simulink library "VIS_LIB"  (Simulink 8.6)
settings: Solver=ode45  StartTime=0.0  StopTime=10.0  RelTol=1e-3
undefined symbols (not defined in the file): AC, SIXOSEM_F_WD_AC_MASTER
libraries: cdsFilt x376, cdsEpicsOut x253, cdsEpicsIn x179, cdsTP x123, VIS_LIB x95, cdsMuxMatrix x91, cdsEpicsStringIn x75, cdsFiltCtrl x72, cdsFunctionCall x70, cdsRms x59, KAGRA_UTIL x25, STATE_BIO_MASTER x5
(part 26 of 38)

== system VIS_LIB/UTILs/OL ==
  note: #DAQ Channels
      |
      | VER_OUT 256
      | HOR_OUT 256
      | SUM_OUT 256
      | CROSS_OUT 256
  SEG1_in : Inport
  SEG2_in : Inport  Port=2
  SEG3_in : Inport  Port=3
  SEG4_in : Inport  Port=4
  CROSS : cdsFilt/Subsystem  Tag=cdsFilt  Description=|
      | Purpose:                                                                                                                                                                                                                                  
      | Standard CDS IIR filter module.                                                                                                                                                                                                           
      |                                                                                                                                                                                                                                           
      | Operation:                                                                                                                                                                                                                                
      | Consists of 10 second order section IIR filters, plus a ramped gain stage. In FE code, also provides pre-defined test points and excitation channel inputs. The filter coefficients are defined in the LIGO system using the 'foton' tool.
      |                                                                                                                                                                                                                                           
      | Usage:                                                                                                                                                                                                                                    
      | Name the part with the desired filter module name.
      settings: AttributesFormatString=%<Tag>
  Demux : Demux
  HOR : cdsFilt/Subsystem  Tag=cdsFilt  Description=|
      | Purpose:                                                                                                                                                                                                                                  
      | Standard CDS IIR filter module.                                                                                                                                                                                                           
      |                                                                                                                                                                                                                                           
      | Operation:                                                                                                                                                                                                                                
      | Consists of 10 second order section IIR filters, plus a ramped gain stage. In FE code, also provides pre-defined test points and excitation channel inputs. The filter coefficients are defined in the LIGO system using the 'foton' tool.
      |                                                                                                                                                                                                                                           
      | Usage:                                                                                                                                                                                                                                    
      | Name the part with the desired filter module name.
      settings: AttributesFormatString=%<Tag>
  MTRX : cdsMuxMatrix/Subsystem  Tag=cdsMuxMatrix  Description=Any size matrix. Inputs and outputs must be connected using Mux and Demux parts.
      settings: AttributesFormatString=%<Tag>
  MTRX_HOR_OUTMON : cdsEpicsOut/Subsystem  Tag=cdsEpicsOutput  Description=|
      | Purpose:                                          
      | Output a FE signal to an EPICS channel.           
      |                                                   
      | Operation:                                        
      | Takes input value and passes it to EPICS record.  
      |                                                   
      | Usage:                                            
      | Name the part with the desired EPICS rrecord name.
      settings: AttributesFormatString=%<Tag>
  MTRX_VER_OUTMON : cdsEpicsOut/Subsystem  Tag=cdsEpicsOutput  Description=|
      | Purpose:                                          
      | Output a FE signal to an EPICS channel.           
      |                                                   
      | Operation:                                        
      | Takes input value and passes it to EPICS record.  
      |                                                   
      | Usage:                                            
      | Name the part with the desired EPICS rrecord name.
      settings: AttributesFormatString=%<Tag>
  Mux : Mux
  PIT_NORM : Product  Inputs=*/
  SEG1 : cdsFilt/Subsystem  Tag=cdsFilt  Description=|
      | Purpose:                                                                                                                                                                                                                                  
      | Standard CDS IIR filter module.                                                                                                                                                                                                           
      |                                                                                                                                                                                                                                           
      | Operation:                                                                                                                                                                                                                                
      | Consists of 10 second order section IIR filters, plus a ramped gain stage. In FE code, also provides pre-defined test points and excitation channel inputs. The filter coefficients are defined in the LIGO system using the 'foton' tool.
      |                                                                                                                                                                                                                                           
      | Usage:                                                                                                                                                                                                                                    
      | Name the part with the desired filter module name.
      settings: AttributesFormatString=%<Tag>
  SEG2 : cdsFilt/Subsystem  Tag=cdsFilt  Description=|
      | Purpose:                                                                                                                                                                                                                                  
      | Standard CDS IIR filter module.                                                                                                                                                                                                           
      |                                                                                                                                                                                                                                           
      | Operation:                                                                                                                                                                                                                                
      | Consists of 10 second order section IIR filters, plus a ramped gain stage. In FE code, also provides pre-defined test points and excitation channel inputs. The filter coefficients are defined in the LIGO system using the 'foton' tool.
      |                                                                                                                                                                                                                                           
      | Usage:                                                                                                                                                                                                                                    
      | Name the part with the desired filter module name.
      settings: AttributesFormatString=%<Tag>
  SEG3 : cdsFilt/Subsystem  Tag=cdsFilt  Description=|
      | Purpose:                                                                                                                                                                                                                                  
      | Standard CDS IIR filter module.                                                                                                                                                                                                           
      |                                                                                                                                                                                                                                           
      | Operation:                                                                                                                                                                                                                                
      | Consists of 10 second order section IIR filters, plus a ramped gain stage. In FE code, also provides pre-defined test points and excitation channel inputs. The filter coefficients are defined in the LIGO system using the 'foton' tool.
      |                                                                                                                                                                                                                                           
      | Usage:                                                                                                                                                                                                                                    
      | Name the part with the desired filter module name.
      settings: AttributesFormatString=%<Tag>
  SEG4 : cdsFilt/Subsystem  Tag=cdsFilt  Description=|
      | Purpose:                                                                                                                                                                                                                                  
      | Standard CDS IIR filter module.                                                                                                                                                                                                           
      |                                                                                                                                                                                                                                           
      | Operation:                                                                                                                                                                                                                                
      | Consists of 10 second order section IIR filters, plus a ramped gain stage. In FE code, also provides pre-defined test points and excitation channel inputs. The filter coefficients are defined in the LIGO system using the 'foton' tool.
      |                                                                                                                                                                                                                                           
      | Usage:                                                                                                                                                                                                                                    
      | Name the part with the desired filter module name.
      settings: AttributesFormatString=%<Tag>
  SUM : cdsFilt/Subsystem  Tag=cdsFilt  Description=|
      | Purpose:                                                                                                                                                                                                                                  
      | Standard CDS IIR filter module.                                                                                                                                                                                                           
      |                                                                                                                                                                                                                                           
      | Operation:                                                                                                                                                                                                                                
      | Consists of 10 second order section IIR filters, plus a ramped gain stage. In FE code, also provides pre-defined test points and excitation channel inputs. The filter coefficients are defined in the LIGO system using the 'foton' tool.
      |                                                                                                                                                                                                                                           
      | Usage:                                                                                                                                                                                                                                    
      | Name the part with the desired filter module name.
      settings: AttributesFormatString=%<Tag>
  Saturation : Saturate  UpperLimit=1e12  LowerLimit=1
  Terminator5 : Terminator
  VER : cdsFilt/Subsystem  Tag=cdsFilt  Description=|
      | Purpose:                                                                                                                                                                                                                                  
      | Standard CDS IIR filter module.                                                                                                                                                                                                           
      |                                                                                                                                                                                                                                           
      | Operation:                                                                                                                                                                                                                                
      | Consists of 10 second order section IIR filters, plus a ramped gain stage. In FE code, also provides pre-defined test points and excitation channel inputs. The filter coefficients are defined in the LIGO system using the 'foton' tool.
      |                                                                                                                                                                                                                                           
      | Usage:                                                                                                                                                                                                                                    
      | Name the part with the desired filter module name.
      settings: AttributesFormatString=%<Tag>
  YAW_NORM : Product  Inputs=*/
  V : Outport
  H : Outport  Port=2
  wires:
  SEG4_in/1 -> SEG4/1
  SEG3_in/1 -> SEG3/1
  SEG1_in/1 -> SEG1/1
  SEG2_in/1 -> SEG2/1
  Mux/1 -> MTRX/1
  MTRX/1 -> Demux/1
  SEG1/1 -> Mux/1
  SEG2/1 -> Mux/2
  SEG3/1 -> Mux/3
  SEG4/1 -> Mux/4
  VER/1 -> V/1
  HOR/1 -> H/1
  SUM/1 -> Saturation/1
  PIT_NORM/1 -> VER/1
  YAW_NORM/1 -> HOR/1
  Demux/1 -> MTRX_VER_OUTMON/1
  Demux/3 -> SUM/1
  Demux/2 -> MTRX_HOR_OUTMON/1
  Saturation/1 -> PIT_NORM/2, YAW_NORM/2
  MTRX_VER_OUTMON/1 -> PIT_NORM/1
  MTRX_HOR_OUTMON/1 -> YAW_NORM/1
  Demux/4 -> CROSS/1
  CROSS/1 -> Terminator5/1

== system VIS_LIB/UTILs/PAY_6DoF ==
  MNL : Inport
  MNT : Inport  Port=2
  MNV : Inport  Port=3
  MNR : Inport  Port=4
  MNP : Inport  Port=5
  MNY : Inport  Port=6
  IML : Inport  Port=7
  IMT : Inport  Port=8
  IMV : Inport  Port=9
  IMR : Inport  Port=10
  IMP : Inport  Port=11
  IMY : Inport  Port=12
  TML : Inport  Port=13
  TMT : Inport  Port=14
  TMV : Inport  Port=15
  TMR : Inport  Port=16
  TMP : Inport  Port=17
  TMY : Inport  Port=18
  IM : VIS_LIB/UTILs/FBs_6DOF
  MN : VIS_LIB/UTILs/FBs_6DOF
  TM : VIS_LIB/UTILs/FBs_6DOF
  MNLo : Outport
  MNTo : Outport  Port=2
  MNVo : Outport  Port=3
  MNRo : Outport  Port=4
  MNPo : Outport  Port=5
  MNYo : Outport  Port=6
  IMLo : Outport  Port=7
  IMTo : Outport  Port=8
  IMVo : Outport  Port=9
  IMRo : Outport  Port=10
  IMPo : Outport  Port=11
  IMYo : Outport  Port=12
  TMLo : Outport  Port=13
  TMTo : Outport  Port=14
  TMVo : Outport  Port=15
  TMRo : Outport  Port=16
  TMPo : Outport  Port=17
  TMYo : Outport  Port=18
  wires:
  TMR/1 -> TM/4
  TMV/1 -> TM/3
  TMT/1 -> TM/2
  TMP/1 -> TM/5
  IMV/1 -> IM/3
  IMP/1 -> IM/5
  IML/1 -> IM/1
  TMY/1 -> TM/6
  IMT/1 -> IM/2
  TML/1 -> TM/1
  MNY/1 -> MN/6
  MNR/1 -> MN/4
  MNP/1 -> MN/5
  MNT/1 -> MN/2
  MNL/1 -> MN/1
  MNV/1 -> MN/3
  IMY/1 -> IM/6
  IMR/1 -> IM/4
  MN/1 -> MNLo/1
  MN/2 -> MNTo/1
  MN/3 -> MNVo/1
  MN/4 -> MNRo/1
  MN/5 -> MNPo/1
  MN/6 -> MNYo/1
  IM/1 -> IMLo/1
  IM/2 -> IMTo/1
  IM/3 -> IMVo/1
  IM/4 -> IMRo/1
  IM/5 -> IMPo/1
  IM/6 -> IMYo/1
  TM/1 -> TMLo/1
  TM/2 -> TMTo/1
  TM/3 -> TMVo/1
  TM/4 -> TMRo/1
  TM/5 -> TMPo/1
  TM/6 -> TMYo/1

== system VIS_LIB/UTILs/PAY_6DoF_DQ ==
  MNL : Inport
  MNT : Inport  Port=2
  MNV : Inport  Port=3
  MNR : Inport  Port=4
  MNP : Inport  Port=5
  MNY : Inport  Port=6
  IML : Inport  Port=7
  IMT : Inport  Port=8
  IMV : Inport  Port=9
  IMR : Inport  Port=10
  IMP : Inport  Port=11
  IMY : Inport  Port=12
  TML : Inport  Port=13
  TMT : Inport  Port=14
  TMV : Inport  Port=15
  TMR : Inport  Port=16
  TMP : Inport  Port=17
  TMY : Inport  Port=18
  IM : VIS_LIB/UTILs/FBs_6DOF_DQ
  MN : VIS_LIB/UTILs/FBs_6DOF_DQ
  TM : VIS_LIB/UTILs/FBs_6DOF_DQ
  MNLo : Outport
  MNTo : Outport  Port=2
  MNVo : Outport  Port=3
  MNRo : Outport  Port=4
  MNPo : Outport  Port=5
  MNYo : Outport  Port=6
  IMLo : Outport  Port=7
  IMTo : Outport  Port=8
  IMVo : Outport  Port=9
  IMRo : Outport  Port=10
  IMPo : Outport  Port=11
  IMYo : Outport  Port=12
  TMLo : Outport  Port=13
  TMTo : Outport  Port=14
  TMVo : Outport  Port=15
  TMRo : Outport  Port=16
  TMPo : Outport  Port=17
  TMYo : Outport  Port=18
  wires:
  TMR/1 -> TM/4
  TMV/1 -> TM/3
  TMT/1 -> TM/2
  TMP/1 -> TM/5
  IMV/1 -> IM/3
  IMP/1 -> IM/5
  IML/1 -> IM/1
  TMY/1 -> TM/6
  IMT/1 -> IM/2
  TML/1 -> TM/1
  MNY/1 -> MN/6
  MNR/1 -> MN/4
  MNP/1 -> MN/5
  MNT/1 -> MN/2
  MNL/1 -> MN/1
  MNV/1 -> MN/3
  IMY/1 -> IM/6
  IMR/1 -> IM/4
  MN/1 -> MNLo/1
  MN/2 -> MNTo/1
  MN/3 -> MNVo/1
  MN/4 -> MNRo/1
  MN/5 -> MNPo/1
  MN/6 -> MNYo/1
  IM/1 -> IMLo/1
  IM/2 -> IMTo/1
  IM/3 -> IMVo/1
  IM/4 -> IMRo/1
  IM/5 -> IMPo/1
  IM/6 -> IMYo/1
  TM/1 -> TMLo/1
  TM/2 -> TMTo/1
  TM/3 -> TMVo/1
  TM/4 -> TMRo/1
  TM/5 -> TMPo/1
  TM/6 -> TMYo/1

== system VIS_LIB/UTILs/PAY_COILs_DQ ==
  MNV1i : Inport
  MNV2i : Inport  Port=2
  MNV3i : Inport  Port=3
  MNH1i : Inport  Port=4
  MNH2i : Inport  Port=5
  MNH3i : Inport  Port=6
  IMV1i : Inport  Port=7
  IMV2i : Inport  Port=8
  IMV3i : Inport  Port=9
  IMH1i : Inport  Port=10
  IMH2i : Inport  Port=11
  IMH3i : Inport  Port=12
  TMH1i : Inport  Port=13
  TMH2i : Inport  Port=14
  TMH3i : Inport  Port=15
  TMH4i : Inport  Port=16
  IM : VIS_LIB/UTILs/6COILs_DQ
  MN : VIS_LIB/UTILs/6COILs_DQ
  TM : VIS_LIB/UTILs/4COILs_DQ
  MNV1 : Outport
  MNV2 : Outport  Port=2
  MNV3 : Outport  Port=3
  MNH1 : Outport  Port=4
  MNH2 : Outport  Port=5
  MNH3 : Outport  Port=6
  IMV1 : Outport  Port=7
  IMV2 : Outport  Port=8
  IMV3 : Outport  Port=9
  IMH1 : Outport  Port=10
  IMH2 : Outport  Port=11
  IMH3 : Outport  Port=12
  TMH1 : Outport  Port=13
  TMH2 : Outport  Port=14
  TMH3 : Outport  Port=15
  TMH4 : Outport  Port=16
  wires:
  TMH2i/1 -> TM/2
  TMH1i/1 -> TM/1
  TMH4i/1 -> TM/4
  MNV1i/1 -> MN/1
  MNV3i/1 -> MN/3
  MNV2i/1 -> MN/2
  IMH3i/1 -> IM/6
  IMH2i/1 -> IM/5
  MNH2i/1 -> MN/5
  TMH3i/1 -> TM/3
  MNH3i/1 -> MN/6
  IMV1i/1 -> IM/1
  MNH1i/1 -> MN/4
  IMV3i/1 -> IM/3
  IMV2i/1 -> IM/2
  IMH1i/1 -> IM/4
  MN/1 -> MNV1/1
  MN/2 -> MNV2/1
  MN/3 -> MNV3/1
  MN/4 -> MNH1/1
  MN/5 -> MNH2/1
  MN/6 -> MNH3/1
  IM/1 -> IMV1/1
  IM/2 -> IMV2/1
  IM/3 -> IMV3/1
  IM/4 -> IMH1/1
  IM/5 -> IMH2/1
  IM/6 -> IMH3/1
  TM/1 -> TMH1/1
  TM/2 -> TMH2/1
  TM/3 -> TMH3/1
  TM/4 -> TMH4/1

== system VIS_LIB/WD2/AC ==
  F0_In : Inport
  SF_In : Inport  Port=2
  BF_In : Inport  Port=3
  BANDLIM : Subsystem
  BFRMS : cdsRms/Subsystem  Tag=cdsRms  Description=|
      | Purpose:
      | Calculate an RMS based on the input signal.
      settings: AttributesFormatString=%<Tag>
  BF_RMS : cdsTP/Subsystem  Tag=Test Point
      settings: AttributesFormatString=%<Tag>
  BF_RMSMON : cdsEpicsOut/Subsystem  Tag=cdsEpicsOutput  Description=|
      | Purpose:                                          
      | Output a FE signal to an EPICS channel.           
      |                                                   
      | Operation:                                        
      | Takes input value and passes it to EPICS record.  
      |                                                   
      | Usage:                                            
      | Name the part with the desired EPICS rrecord name.
      settings: AttributesFormatString=%<Tag>
  F0RMS : cdsRms/Subsystem  Tag=cdsRms  Description=|
      | Purpose:
      | Calculate an RMS based on the input signal.
      settings: AttributesFormatString=%<Tag>
  F0_RMS : cdsTP/Subsystem  Tag=Test Point
      settings: AttributesFormatString=%<Tag>
  F0_RMSMON : cdsEpicsOut/Subsystem  Tag=cdsEpicsOutput  Description=|
      | Purpose:                                          
      | Output a FE signal to an EPICS channel.           
      |                                                   
      | Operation:                                        
      | Takes input value and passes it to EPICS record.  
      |                                                   
      | Usage:                                            
      | Name the part with the desired EPICS rrecord name.
      settings: AttributesFormatString=%<Tag>
  Operator1 : RelationalOperator  Operator=>  OutDataTypeStr=boolean
  Operator2 : RelationalOperator  Operator=>  OutDataTypeStr=boolean
  Operator3 : RelationalOperator  Operator=>  OutDataTypeStr=boolean
  RMS_MAX : cdsEpicsIn/Subsystem  Tag=cdsEpicsIn  Description=|
      | Purpose:                                                                              
      | Create an EPICS input channel connection to the FE realtime controls.                 
      |                                                                                       
      | Operation:                                                                            
      | Outputs value from an EPICS ai record. Value is floating point with a precision of 3..
      |                                                                                       
      | Usage:                                                                                
      | Name the part with the desired EPICS channel name.
      settings: AttributesFormatString=%<Tag>
  SFRMS : cdsRms/Subsystem  Tag=cdsRms  Description=|
      | Purpose:
      | Calculate an RMS based on the input signal.
      settings: AttributesFormatString=%<Tag>
  SF_RMS : cdsTP/Subsystem  Tag=Test Point
      settings: AttributesFormatString=%<Tag>
  SF_RMSMON : cdsEpicsOut/Subsystem  Tag=cdsEpicsOutput  Description=|
      | Purpose:                                          
      | Output a FE signal to an EPICS channel.           
      |                                                   
      | Operation:                                        
      | Takes input value and passes it to EPICS record.  
      |                                                   
      | Usage:                                            
      | Name the part with the desired EPICS rrecord name.
      settings: AttributesFormatString=%<Tag>
  Sum1 : Sum  Inputs=+++
  FLAG : Outport
  wires:
  BANDLIM/3(BF_Out) -> BFRMS/1
  BF_In/1 -> BANDLIM/3(BF_In)
  F0RMS/1 -> F0_RMS/1, F0_RMSMON/1
  F0_RMSMON/1 -> Operator1/1
  SF_In/1 -> BANDLIM/2(SF_In)
  F0_In/1 -> BANDLIM/1(F0_In)
  SFRMS/1 -> SF_RMS/1, SF_RMSMON/1
  SF_RMSMON/1 -> Operator2/1
  BFRMS/1 -> BF_RMS/1, BF_RMSMON/1
  BF_RMSMON/1 -> Operator3/1
  BANDLIM/2(SF_Out) -> SFRMS/1
  BANDLIM/1(F0_Out) -> F0RMS/1
  RMS_MAX/1 -> Operator3/2, Operator2/2, Operator1/2
  Operator3/1 -> Sum1/3
  Operator2/1 -> Sum1/2
  Operator1/1 -> Sum1/1
  Sum1/1 -> FLAG/1

== system VIS_LIB/WD3/OSEMAC ==
  V1_In : Inport
  V2_In : Inport  Port=2
  V3_In : Inport  Port=3
  H1_In : Inport  Port=4
  H2_In1 : Inport  Port=5
  H3_In1 : Inport  Port=6
  BANDLIM : Subsystem
  H1RMS : cdsRms/Subsystem  Tag=cdsRms  Description=|
      | Purpose:
      | Calculate an RMS based on the input signal.
      settings: AttributesFormatString=%<Tag>
  H1_RMS : cdsTP/Subsystem  Tag=Test Point
      settings: AttributesFormatString=%<Tag>
  H1_RMSMON : cdsEpicsOut/Subsystem  Tag=cdsEpicsOutput  Description=|
      | Purpose:                                          
      | Output a FE signal to an EPICS channel.           
      |                                                   
      | Operation:                                        
      | Takes input value and passes it to EPICS record.  
      |                                                   
      | Usage:                                            
      | Name the part with the desired EPICS rrecord name.
      settings: AttributesFormatString=%<Tag>
  H2RMS : cdsRms/Subsystem  Tag=cdsRms  Description=|
      | Purpose:
      | Calculate an RMS based on the input signal.
      settings: AttributesFormatString=%<Tag>
  H2_RMS : cdsTP/Subsystem  Tag=Test Point
      settings: AttributesFormatString=%<Tag>
  H2_RMSMON : cdsEpicsOut/Subsystem  Tag=cdsEpicsOutput  Description=|
      | Purpose:                                          
      | Output a FE signal to an EPICS channel.           
      |                                                   
      | Operation:                                        
      | Takes input value and passes it to EPICS record.  
      |                                                   
      | Usage:                                            
      | Name the part with the desired EPICS rrecord name.
      settings: AttributesFormatString=%<Tag>
  H3RMS : cdsRms/Subsystem  Tag=cdsRms  Description=|
      | Purpose:
      | Calculate an RMS based on the input signal.
      settings: AttributesFormatString=%<Tag>
  H3_RMS : cdsTP/Subsystem  Tag=Test Point
      settings: AttributesFormatString=%<Tag>
  H3_RMSMON : cdsEpicsOut/Subsystem  Tag=cdsEpicsOutput  Description=|
      | Purpose:                                          
      | Output a FE signal to an EPICS channel.           
      |                                                   
      | Operation:                                        
      | Takes input value and passes it to EPICS record.  
      |                                                   
      | Usage:                                            
      | Name the part with the desired EPICS rrecord name.
      settings: AttributesFormatString=%<Tag>
  Operator{1,3..6} (5 alike) : RelationalOperator  Operator=>  OutDataTypeStr=boolean
  Operator2 : RelationalOperator  Operator=>  OutDataTypeStr=boolean  ZeroCross=off
  RMS_MAX : cdsEpicsIn/Subsystem  Tag=cdsEpicsIn  Description=|
      | Purpose:                                                                              
      | Create an EPICS input channel connection to the FE realtime controls.                 
      |                                                                                       
      | Operation:                                                                            
      | Outputs value from an EPICS ai record. Value is floating point with a precision of 3..
      |                                                                                       
      | Usage:                                                                                
      | Name the part with the desired EPICS channel name.
      settings: AttributesFormatString=%<Tag>
  Sum1 : Sum  Inputs=++++++
  V1RMS : cdsRms/Subsystem  Tag=cdsRms  Description=|
      | Purpose:
      | Calculate an RMS based on the input signal.
      settings: AttributesFormatString=%<Tag>
  V1_RMS : cdsTP/Subsystem  Tag=Test Point
      settings: AttributesFormatString=%<Tag>
  V1_RMSMON : cdsEpicsOut/Subsystem  Tag=cdsEpicsOutput  Description=|
      | Purpose:                                          
      | Output a FE signal to an EPICS channel.           
      |                                                   
      | Operation:                                        
      | Takes input value and passes it to EPICS record.  
      |                                                   
      | Usage:                                            
      | Name the part with the desired EPICS rrecord name.
      settings: AttributesFormatString=%<Tag>
  V2RMS : cdsRms/Subsystem  Tag=cdsRms  Description=|
      | Purpose:
      | Calculate an RMS based on the input signal.
      settings: AttributesFormatString=%<Tag>
  V2_RMS : cdsTP/Subsystem  Tag=Test Point
      settings: AttributesFormatString=%<Tag>
  V2_RMSMON : cdsEpicsOut/Subsystem  Tag=cdsEpicsOutput  Description=|
      | Purpose:                                          
      | Output a FE signal to an EPICS channel.           
      |                                                   
      | Operation:                                        
      | Takes input value and passes it to EPICS record.  
      |                                                   
      | Usage:                                            
      | Name the part with the desired EPICS rrecord name.
      settings: AttributesFormatString=%<Tag>
  V3RMS : cdsRms/Subsystem  Tag=cdsRms  Description=|
      | Purpose:
      | Calculate an RMS based on the input signal.
      settings: AttributesFormatString=%<Tag>
  V3_RMS : cdsTP/Subsystem  Tag=Test Point
      settings: AttributesFormatString=%<Tag>
  V3_RMSMON : cdsEpicsOut/Subsystem  Tag=cdsEpicsOutput  Description=|
      | Purpose:                                          
      | Output a FE signal to an EPICS channel.           
      |                                                   
      | Operation:                                        
      | Takes input value and passes it to EPICS record.  
      |                                                   
      | Usage:                                            
      | Name the part with the desired EPICS rrecord name.
      settings: AttributesFormatString=%<Tag>
  FLAG : Outport
  wires:
  BANDLIM/6(H3_Out) -> H3RMS/1
  BANDLIM/5(H2_Out) -> H2RMS/1
  BANDLIM/4(H1_Out) -> H1RMS/1
  BANDLIM/3(V3_Out) -> V3RMS/1
  BANDLIM/2(V2_Out) -> V2RMS/1
  BANDLIM/1(V1_Out) -> V1RMS/1
  H3_In1/1 -> BANDLIM/6(H3_In)
  H2_In1/1 -> BANDLIM/5(H2_In)
  H1_In/1 -> BANDLIM/4(H1_In)
  V3_In/1 -> BANDLIM/3(V3_In)
  V2_In/1 -> BANDLIM/2(V2_In)
  V1_In/1 -> BANDLIM/1(V1_In)
  Operator1/1 -> Sum1/1
  Operator2/1 -> Sum1/2
  Operator3/1 -> Sum1/3
  Operator4/1 -> Sum1/4
  RMS_MAX/1 -> Operator1/2, Operator2/2, Operator3/2, Operator4/2, Operator5/2, Operator6/2
  V2RMS/1 -> V2_RMS/1, V2_RMSMON/1
  V1RMS/1 -> V1_RMS/1, V1_RMSMON/1
  V3RMS/1 -> V3_RMS/1, V3_RMSMON/1
  H1RMS/1 -> H1_RMS/1, H1_RMSMON/1
  Sum1/1 -> FLAG/1
  H2RMS/1 -> H2_RMS/1, H2_RMSMON/1
  H3RMS/1 -> H3_RMS/1, H3_RMSMON/1
  V1_RMSMON/1 -> Operator1/1
  V2_RMSMON/1 -> Operator2/1
  V3_RMSMON/1 -> Operator3/1
  H1_RMSMON/1 -> Operator4/1
  H2_RMSMON/1 -> Operator5/1
  H3_RMSMON/1 -> Operator6/1
  Operator5/1 -> Sum1/5
  Operator6/1 -> Sum1/6

== system VIS_LIB/WD4/AC ==
  SF_In : Inport
  BF_In : Inport  Port=2
  BANDLIM : Subsystem
  BFRMS : cdsRms/Subsystem  Tag=cdsRms  Description=|
      | Purpose:
      | Calculate an RMS based on the input signal.
      settings: AttributesFormatString=%<Tag>
  BF_RMS : cdsTP/Subsystem  Tag=Test Point
      settings: AttributesFormatString=%<Tag>
  BF_RMSMON : cdsEpicsOut/Subsystem  Tag=cdsEpicsOutput  Description=|
      | Purpose:                                          
      | Output a FE signal to an EPICS channel.           
      |                                                   
      | Operation:                                        
      | Takes input value and passes it to EPICS record.  
      |                                                   
      | Usage:                                            
      | Name the part with the desired EPICS rrecord name.
      settings: AttributesFormatString=%<Tag>
  Operator2 : RelationalOperator  Operator=>  OutDataTypeStr=boolean
  Operator3 : RelationalOperator  Operator=>  OutDataTypeStr=boolean
  RMS_MAX : cdsEpicsIn/Subsystem  Tag=cdsEpicsIn  Description=|
      | Purpose:                                                                              
      | Create an EPICS input channel connection to the FE realtime controls.                 
      |                                                                                       
      | Operation:                                                                            
      | Outputs value from an EPICS ai record. Value is floating point with a precision of 3..
      |                                                                                       
      | Usage:                                                                                
      | Name the part with the desired EPICS channel name.
      settings: AttributesFormatString=%<Tag>
  SFRMS : cdsRms/Subsystem  Tag=cdsRms  Description=|
      | Purpose:
      | Calculate an RMS based on the input signal.
      settings: AttributesFormatString=%<Tag>
  SF_RMS : cdsTP/Subsystem  Tag=Test Point
      settings: AttributesFormatString=%<Tag>
  SF_RMSMON : cdsEpicsOut/Subsystem  Tag=cdsEpicsOutput  Description=|
      | Purpose:                                          
      | Output a FE signal to an EPICS channel.           
      |                                                   
      | Operation:                                        
      | Takes input value and passes it to EPICS record.  
      |                                                   
      | Usage:                                            
      | Name the part with the desired EPICS rrecord name.
      settings: AttributesFormatString=%<Tag>
  Sum1 : Sum
  FLAG : Outport
  wires:
  BANDLIM/2(BF_Out) -> BFRMS/1
  BF_In/1 -> BANDLIM/2(BF_In)
  SF_In/1 -> BANDLIM/1(SF_In)
  SFRMS/1 -> SF_RMS/1, SF_RMSMON/1
  SF_RMSMON/1 -> Operator2/1
  BFRMS/1 -> BF_RMS/1, BF_RMSMON/1
  BF_RMSMON/1 -> Operator3/1
  BANDLIM/1(SF_Out) -> SFRMS/1
  RMS_MAX/1 -> Operator3/2, Operator2/2
  Operator3/1 -> Sum1/2
  Sum1/1 -> FLAG/1
  Operator2/1 -> Sum1/1

== system VIS_LIB/CRYp Blocks/PSWD/PSAC ==
  V1_In : Inport
  V2_In : Inport  Port=2
  V3_In : Inport  Port=3
  H1_In : Inport  Port=4
  H2_In1 : Inport  Port=5
  H3_In1 : Inport  Port=6
  BANDLIM : Subsystem
  H1RMS : cdsRms/Subsystem  Tag=cdsRms  Description=|
      | Purpose:
      | Calculate an RMS based on the input signal.
      settings: AttributesFormatString=%<Tag>
  H1_RMS : cdsTP/Subsystem  Tag=Test Point
      settings: AttributesFormatString=%<Tag>
  H1_RMSMON : cdsEpicsOut/Subsystem  Tag=cdsEpicsOutput  Description=|
      | Purpose:                                          
      | Output a FE signal to an EPICS channel.           
      |                                                   
      | Operation:                                        
      | Takes input value and passes it to EPICS record.  
      |                                                   
      | Usage:                                            
      | Name the part with the desired EPICS rrecord name.
      settings: AttributesFormatString=%<Tag>
  H2RMS : cdsRms/Subsystem  Tag=cdsRms  Description=|
      | Purpose:
      | Calculate an RMS based on the input signal.
      settings: AttributesFormatString=%<Tag>
  H2_RMS : cdsTP/Subsystem  Tag=Test Point
      settings: AttributesFormatString=%<Tag>
  H2_RMSMON : cdsEpicsOut/Subsystem  Tag=cdsEpicsOutput  Description=|
      | Purpose:                                          
      | Output a FE signal to an EPICS channel.           
      |                                                   
      | Operation:                                        
      | Takes input value and passes it to EPICS record.  
      |                                                   
      | Usage:                                            
      | Name the part with the desired EPICS rrecord name.
      settings: AttributesFormatString=%<Tag>
  H3RMS : cdsRms/Subsystem  Tag=cdsRms  Description=|
      | Purpose:
      | Calculate an RMS based on the input signal.
      settings: AttributesFormatString=%<Tag>
  H3_RMS : cdsTP/Subsystem  Tag=Test Point
      settings: AttributesFormatString=%<Tag>
  H3_RMSMON : cdsEpicsOut/Subsystem  Tag=cdsEpicsOutput  Description=|
      | Purpose:                                          
      | Output a FE signal to an EPICS channel.           
      |                                                   
      | Operation:                                        
      | Takes input value and passes it to EPICS record.  
      |                                                   
      | Usage:                                            
      | Name the part with the desired EPICS rrecord name.
      settings: AttributesFormatString=%<Tag>
  Operator{1,3..6} (5 alike) : RelationalOperator  Operator=>  OutDataTypeStr=boolean
  Operator2 : RelationalOperator  Operator=>  OutDataTypeStr=boolean  ZeroCross=off
  RMS_MAX : cdsEpicsIn/Subsystem  Tag=cdsEpicsIn  Description=|
      | Purpose:                                                                              
      | Create an EPICS input channel connection to the FE realtime controls.                 
      |                                                                                       
      | Operation:                                                                            
      | Outputs value from an EPICS ai record. Value is floating point with a precision of 3..
      |                                                                                       
      | Usage:                                                                                
      | Name the part with the desired EPICS channel name.
      settings: AttributesFormatString=%<Tag>
  Sum1 : Sum  Inputs=++++++
  V1RMS : cdsRms/Subsystem  Tag=cdsRms  Description=|
      | Purpose:
      | Calculate an RMS based on the input signal.
      settings: AttributesFormatString=%<Tag>
  V1_RMS : cdsTP/Subsystem  Tag=Test Point
      settings: AttributesFormatString=%<Tag>
  V1_RMSMON : cdsEpicsOut/Subsystem  Tag=cdsEpicsOutput  Description=|
      | Purpose:                                          
      | Output a FE signal to an EPICS channel.           
      |                                                   
      | Operation:                                        
      | Takes input value and passes it to EPICS record.  
      |                                                   
      | Usage:                                            
      | Name the part with the desired EPICS rrecord name.
      settings: AttributesFormatString=%<Tag>
  V2RMS : cdsRms/Subsystem  Tag=cdsRms  Description=|
      | Purpose:
      | Calculate an RMS based on the input signal.
      settings: AttributesFormatString=%<Tag>
  V2_RMS : cdsTP/Subsystem  Tag=Test Point
      settings: AttributesFormatString=%<Tag>
  V2_RMSMON : cdsEpicsOut/Subsystem  Tag=cdsEpicsOutput  Description=|
      | Purpose:                                          
      | Output a FE signal to an EPICS channel.           
      |                                                   
      | Operation:                                        
      | Takes input value and passes it to EPICS record.  
      |                                                   
      | Usage:                                            
      | Name the part with the desired EPICS rrecord name.
      settings: AttributesFormatString=%<Tag>
  V3RMS : cdsRms/Subsystem  Tag=cdsRms  Description=|
      | Purpose:
      | Calculate an RMS based on the input signal.
      settings: AttributesFormatString=%<Tag>
  V3_RMS : cdsTP/Subsystem  Tag=Test Point
      settings: AttributesFormatString=%<Tag>
  V3_RMSMON : cdsEpicsOut/Subsystem  Tag=cdsEpicsOutput  Description=|
      | Purpose:                                          
      | Output a FE signal to an EPICS channel.           
      |                                                   
      | Operation:                                        
      | Takes input value and passes it to EPICS record.  
      |                                                   
      | Usage:                                            
      | Name the part with the desired EPICS rrecord name.
      settings: AttributesFormatString=%<Tag>
  FLAG : Outport
  wires:
  BANDLIM/6(H3_Out) -> H3RMS/1
  BANDLIM/5(H2_Out) -> H2RMS/1
  BANDLIM/4(H1_Out) -> H1RMS/1
  BANDLIM/3(V3_Out) -> V3RMS/1
  BANDLIM/2(V2_Out) -> V2RMS/1
  BANDLIM/1(V1_Out) -> V1RMS/1
  H3_In1/1 -> BANDLIM/6(H3_In)
  H2_In1/1 -> BANDLIM/5(H2_In)
  H1_In/1 -> BANDLIM/4(H1_In)
  V3_In/1 -> BANDLIM/3(V3_In)
  V2_In/1 -> BANDLIM/2(V2_In)
  V1_In/1 -> BANDLIM/1(V1_In)
  Operator1/1 -> Sum1/1
  Operator2/1 -> Sum1/2
  Operator3/1 -> Sum1/3
  Operator4/1 -> Sum1/4
  RMS_MAX/1 -> Operator1/2, Operator2/2, Operator3/2, Operator4/2, Operator5/2, Operator6/2
  V2RMS/1 -> V2_RMS/1, V2_RMSMON/1
  V1RMS/1 -> V1_RMS/1, V1_RMSMON/1
  V3RMS/1 -> V3_RMS/1, V3_RMSMON/1
  H1RMS/1 -> H1_RMS/1, H1_RMSMON/1
  Sum1/1 -> FLAG/1
  H2RMS/1 -> H2_RMS/1, H2_RMSMON/1
  H3RMS/1 -> H3_RMS/1, H3_RMSMON/1
  V1_RMSMON/1 -> Operator1/1
  V2_RMSMON/1 -> Operator2/1
  V3_RMSMON/1 -> Operator3/1
  H1_RMSMON/1 -> Operator4/1
  H2_RMSMON/1 -> Operator5/1
  H3_RMSMON/1 -> Operator6/1
  Operator5/1 -> Sum1/5
  Operator6/1 -> Sum1/6
